simulink model "end_sem_mimuro_plot"  (R2023b)
settings: Solver=FixedStepAuto  StartTime=0.0  StopTime=20  FixedStep=0.001  RelTol=1e-3
undefined symbols (not defined in the file): simscape, X, Y, Z
libraries: sm_lib x108, nesl_utility x77, fl_lib x23, sdl_lib x5, sharedtransform x4
(part 4 of 6)

== system end_sem_mimuro_plot/Tire RL ==
  Cylindrical Solid : sm_lib/Body Elements/Cylindrical Solid  Commented=on  GraphicAmbientColor=[0.15 0.15 0.15 1.0]  BasedOnType=Density  CenterOfMass=[0 0 0]  CenterOfMassUnits=m  GraphicDiffuseColor=[0.5 0.5 0.5]  CylinderLength=0.21  CylinderLengthUnits=m  CylinderRadius=0.345  CylinderRadiusUnits=m  Density=1000  DensityUnits=kg/m^3  DoExposeReferenceFrame=on  GraphicEmissiveColor=[0.0 0.0 0.0 1.0]  ExportEntireGeometry=off  SerializedFrames=<Frames/>  MarkerShape=Sphere  MarkerSize=10  GraphicType=FromGeometry  InertiaType=Custom  Mass=20  MassUnits=kg  MomentsOfInertia=[1 2 1]  MomentsOfInertiaUnits=kg*m^2  GraphicOpacity=1.0  ProductsOfInertia=[0 0 0]  ProductsOfInertiaUnits=kg*m^2  GraphicShininess=75  GraphicSpecularColor=[0.5 0.5 0.5 1.0]  GraphicVisPropType=SimpleVisualProperties
  Inertia : sm_lib/Body Elements/Inertia  InertiaType=Custom  Mass=20  MassUnits=kg  CenterOfMass=[0 0 0]  CenterOfMassUnits=m  MomentsOfInertia=[1 2 1]  MomentsOfInertiaUnits=kg*m^2  ProductsOfInertia=[0 0 0]  ProductsOfInertiaUnits=kg*m^2  GraphicType=Marker  MarkerShape=Frame  MarkerSize=50  GraphicVisPropType=SimpleVisualProperties  GraphicDiffuseColor=[1 1 0.06667]  GraphicSpecularColor=[0.5 0.5 0.5 1.0]  GraphicAmbientColor=[0.15 0.15 0.15 1.0]  GraphicEmissiveColor=[0.0 0.0 0.0 1.0]  GraphicShininess=75  GraphicOpacity=1.0
  Tire : sm_lib/Forces and Torques/Magic Formula Tire Force and Torque  TireSide=Left  TireParameters=simscape.multibody.tirread('sm_car_heave_roll_tire_245_60_R16.tir')  SlipMode=Combined  NumericParameters=[0.1 0.1 0.1 0.1 5.0 1e-4 1e-4 1e-7 1e-7 1e-4 1e-4 0.1 1e-4 1e-4 1e-4 1e-4 1e-4 1e-4 1e-4 1e-4 1e-4]  ScalingCoefficientLMUXMode=FromTireParameters  ScalingCoefficientLMUYMode=FromTireParameters  SenseContactSignal=off  TireWrenchFrame=ContactFrame  SenseTireForce=off  SenseTireTorque=off  SensePneumaticTrail=off  SenseLongitudinalSlip=off  SenseSaturatedLongitudinalSlip=off  SenseSlipAngle=off  SenseSaturatedSlipAngle=off  SenseTurnSlip=off  SenseRelativeLongitudinalVelocity=off  SenseRelativeLateralVelocity=off  SenseLongitudinalSlipVelocity=off  SenseLateralSlipVelocity=off  SenseYawVelocity=off  SenseCamberAngle=off  SenseSaturatedCamberAngle=off  SenseCamberVelocity=off  SenseSpinVelocity=off  SenseFreeRadius=off  SenseLoadedRadius=off  SenseEffectiveRollingRadius=off  SenseLongitudinalFrictionCoefficient=off  SenseLateralFrictionCoefficient=off  SenseContactBaseRotation=off  SenseContactBaseTranslation=off  SenseContactFollowerRotation=off  SenseContactFollowerTranslation=off
  Tire Visual : Subsystem  mask(Tire Visual){tireWidth=245, aspectRatio=60, rimDia=16, rimWidth=0.205, box_color=[0.2,0.2,0.2], pulley_clr=[199,182,123]/255, box_opc=1, pulley_opc=1, lr=Left, b=9, ir=0.1, hr=0.035}
      mask prompts: rimWidth "Rim width (m)"; box_color "Tire color"; pulley_clr "Rim Color"; box_opc "Tire opacity"; pulley_opc "Rim opacity"; lr "Left/Right"; b "No. of spokes"; ir "Inner radius (m)"; hr "Hole radius (m)"
      mask init: same as end_sem_mimuro_plot/Tire FL/Tire Visual
      mask TypeOptions lr: Left | Right
      mask DialogControl ParameterGroupVar Prompt: Tire size
      mask DialogControl Control2 Prompt: /
      mask DialogControl Control3 Prompt: R
      mask DialogControl Container3 Prompt: Visual appearance
      mask DialogControl Container4 Prompt: Rim
      mask Display:
      | try
      |     image('wheel_no_brake.png')
      | catch ME
      |     fprintf('TireVisual\n')
      | end
      | 
      | % text(5,90,'Parametric Wheel Visual')
      | % f = 60;
      | % fx = 70;
      | % fx0 = 25;
      | % fy = 70;
      | % fy0 = 10;
      | % plot(-fx0+fx.*[0.8828 0.8769 0.8597 0.7299 0.7043 0.6745 0.6443 0.6195 0.5884 0.5712 0.5653 0.5573 0.5346 0.4985 0.4515 0.3965 0.3373 ]+160/2-0.43*f,-fy0+fy.*[0.3654 0.3482 0.3335 0.2583 0.2486 0.2453 0.2486 0.2583 0.2764 0.2911 0.3083 0.2449 0.1945 0.1609 0.1462 0.1520 0.1768 ]+0.3*f)
      | % plot(-fx0+fx.*[0.3255 0.3889 0.3965 0.4112 0.4313 0.3767 ]+160/2-0.43*f,-fy0+fy.*[0.1491 0.1222 0.1520 0.1777 0.1949 0.2184 ]+0.3*f)
      | % plot(-fx0+fx.*[0.3553 0.4112 0.4633 0.4826 0.5464 ]+160/2-0.43*f,-fy0+fy.*[0.2012 0.1777 0.1722 0.1898 0.2268 ]+0.3*f)
      | % plot(-fx0+fx.*[0.5426 0.5262 0.4826 0.4313 0.5603 0.5603 0.5065 ]+160/2-0.43*f,-fy0+fy.*[0.2184 0.2037 0.1898 0.1949 0.2692 0.2701 0.2932 ]+0.3*f)
      | % plot(-fx0+fx.*[0.5279 0.5460 0.4868 ]+160/2-0.43*f,-fy0+fy.*[0.3007 0.2969 0.3402 ]+0.3*f)
      | % plot(-fx0+fx.*[0.5279 0.5624 ]+160/2-0.43*f,-fy0+fy.*[0.3007 0.2856 ]+0.3*f)
      | % plot(-fx0+fx.*[0.5628 0.5460 ]+160/2-0.43*f,-fy0+fy.*[0.2898 0.2969 ]+0.3*f)
      | % plot(-fx0+fx.*[0.5712 0.5628 0.5573 ]+160/2-0.43*f,-fy0+fy.*[0.2911 0.2222 0.2449 ]+0.3*f)
      | % plot(-fx0+fx.*[0.5586 0.5422 0.5082 0.4633 0.4515 0.4481 0.3889 0.3902 0.4544 0.5099 0.5523 0.5792 0.5884 ]+160/2-0.43*f,-fy0+fy.*[0.2541 0.2180 0.1861 0.1722 0.1462 0.1163 0.1222 0.0928 0.0865 0.1033 0.1428 0.2016 0.2764 ]+0.3*f)
      | % plot(-fx0+fx.*[0.6195 0.6090 0.5792 0.5628 0.5380 0.5346 0.5422 ]+160/2-0.43*f,-fy0+fy.*[0.2583 0.1751 0.2016 0.2222 0.1680 0.1945 0.2180 ]+0.3*f)
      | % plot(-fx0+fx.*[0.5262 0.5082 0.4985 0.4994 0.5380 0.5523 0.5792 0.6090 0.6333 0.6443 ]+160/2-0.43*f,-fy0+fy.*[0.2037 0.1861 0.1609 0.1319 0.1680 0.1428 0.1092 0.1751 0.1596 0.2486 ]+0.3*f)
      | % plot(-fx0+fx.*[0.6745 0.6627 0.6333 0.6018 0.5792 0.5317 0.5099 0.4994 0.4481 0.4544 0.4700 0.5317 0.5510 0.6018 0.6291 0.6627 0.6926 0.7043 ]+160/2-0.43*f,-fy0+fy.*[0.2453 0.1508 0.1596 0.0890 0.1092 0.0655 0.1033 0.1319 0.1163 0.0865 0.0462 0.0655 0.0416 0.0890 0.0764 0.1508 0.1508 0.2486 ]+0.3*f)
      | % plot(-fx0+fx.*[0.7299 0.7178 0.6926 0.6577 0.6291 0.5758 0.5510 0.4851 0.4700 0.3986 0.3213 0.2440 0.1718 0.1100 0.0626 ]+160/2-0.43*f,-fy0+fy.*[0.2583 0.1596 0.1508 0.0739 0.0764 0.0269 0.0416 0.0210 0.0462 0.0533 0.0861 0.1424 0.2184 0.3087 0.4074 ]+0.3*f)
      | % plot(-fx0+fx.*[0.0487 0.0995 0.1100 0.1323 0.1516 0.1760 0.1399 ]+160/2-0.43*f,-fy0+fy.*[0.4082 0.3028 0.3087 0.3213 0.3326 0.3469 0.4221 ]+0.3*f)
      | % plot(-fx0+fx.*[0.1126 0.1516 0.2024 0.2234 0.2474 0.2709 0.4011 0.4200 0.4322 0.3847 0.3486 0.3255 ]+160/2-0.43*f,-fy0+fy.*[0.4141 0.3326 0.2579 0.2776 0.2969 0.3121 0.3872 0.3965 0.3982 0.4670 0.5426 0.6191 ]+0.3*f)
      | % plot(-fx0+fx.*[0.3486 0.3410 0.3755 0.3847 ]+160/2-0.43*f,-fy0+fy.*[0.5426 0.5330 0.4616 0.4670 ]+0.3*f)
      | % plot(-fx0+fx.*[0.3755 0.3570 0.3234 ]+160/2-0.43*f,-fy0+fy.*[0.4616 0.4511 0.5212 ]+0.3*f)
      | % plot(-fx0+fx.*[0.3570 0.2272 0.1936 ]+160/2-0.43*f,-fy0+fy.*[0.4511 0.3759 0.4460 ]+0.3*f)
      | % plot(-fx0+fx.*[0.1684 0.2029 0.2272 0.2709 0.3217 0.4519 0.4721 0.4868 0.4322 ]+160/2-0.43*f,-fy0+fy.*[0.4334 0.3625 0.3759 0.3121 0.2583 0.3331 0.3415 0.3402 0.3982 ]+0.3*f)
      | % plot(-fx0+fx.*[0.4200 0.3755 ]+160/2-0.43*f,-fy0+fy.*[0.3965 0.4616 ]+0.3*f)
      | % plot(-fx0+fx.*[0.3570 0.4011 0.4519 0.5065 0.5279 0.4721 0.4200 ]+160/2-0.43*f,-fy0+fy.*[0.4511 0.3872 0.3331 0.2932 0.3007 0.3415 0.3965 ]+0.3*f)
      | % plot(-fx0+fx.*[0.5065 0.3767 0.3217 0.2995 0.2474 0.2029 0.1760 0.2234 0.2785 0.2995 0.3553 0.3767 ]+160/2-0.43*f,-fy0+fy.*[0.2932 0.2184 0.2583 0.2419 0.2969 0.3625 0.3469 0.2776 0.2197 0.2419 0.2012 0.2184 ]+0.3*f)
      | % plot(-fx0+fx.*[0.3553 0.3373 0.2785 0.2617 0.2024 0.1873 0.1323 0.0899 0.0630 0.0542 0.0231 0.0059 0.0000 0.0113 0.0168 0.0332 0.0630 0.0878 0.1172 0.1470 0.1722 0.3024 0.3192 0.3255 0.3179 0.3121 0.2948 0.1651 0.1394 0.1470 0.1172 0.0878 0.0630 0.0332 0.0168 0.0113 0.0000 ]+160/2-0.43*f,-fy0+fy.*[0.2012 0.1768 0.2197 0.1957 0.2579 0.2402 0.3213 0.4099 0.4994 0.5846 0.6027 0.6174 0.6346 0.5271 0.5157 0.5078 0.4994 0.4964 0.4990 0.5061 0.5174 0.5922 0.6056 0.6191 0.6917 0.6745 0.6598 0.5846 0.5745 0.6350 0.6350 0.6434 0.6594 0.6858 0.7064 0.7291 0.6346 ]+0.3*f)
      | % plot(-fx0+fx.*[0.0059 0.0168 ]+160/2-0.43*f,-fy0+fy.*[0.6174 0.7064 ]+0.3*f)
      | % plot(-fx0+fx.*[0.0113 0.0454 0.0529 0.0181 0.0113 ]+160/2-0.43*f,-fy0+fy.*[0.7291 0.8034 0.8270 0.7497 0.7291 ]+0.3*f)
      | % plot(-fx0+fx.*[0.0168 0.0487 0.0454 ]+160/2-0.43*f,-fy0+fy.*[0.7064 0.7770 0.8034 ]+0.3*f)
      | % plot(-fx0+fx.*[0.0487 0.0626 0.0899 0.0630 0.0542 0.0794 0.0878 0.1126 0.0899 ]+160/2-0.43*f,-fy0+fy.*[0.7770 0.7518 0.7182 0.6594 0.5846 0.5745 0.6434 0.6976 0.7182 ]+0.3*f)
      | % plot(-fx0+fx.*[0.1126 0.1399 0.1684 0.1936 0.2570 ]+160/2-0.43*f,-fy0+fy.*[0.6976 0.6854 0.6829 0.6905 0.7274 ]+0.3*f)
      | % plot(-fx0+fx.*[0.3011 0.1722 0.1936 ]+160/2-0.43*f,-fy0+fy.*[0.7182 0.6438 0.6905 ]+0.3*f)
      | % plot(-fx0+fx.*[0.1684 0.1470 0.1722 0.1651 0.1722 0.1936 0.3234 0.3410 0.3192 0.3121 0.3163 ]+160/2-0.43*f,-fy0+fy.*[0.6829 0.6350 0.6438 0.5846 0.5174 0.4460 0.5212 0.5330 0.6056 0.6745 0.7119 ]+0.3*f)
      | % plot(-fx0+fx.*[0.3200 0.3179 ]+160/2-0.43*f,-fy0+fy.*[0.7102 0.6917 ]+0.3*f)
      | % plot(-fx0+fx.*[0.3020 0.2948 0.3024 0.3234 ]+160/2-0.43*f,-fy0+fy.*[0.7178 0.6598 0.5922 0.5212 ]+0.3*f)
      | % plot(-fx0+fx.*[0.1470 0.1394 0.1096 0.1172 0.1399 0.1760 0.1516 0.1323 0.1100 0.0995 0.0987 0.1688 0.1806 0.1999 0.3297 0.2566 0.1264 0.0701 0.0529 0.1084 0.1264 0.1999 ]+160/2-0.43*f,-fy0+fy.*[0.5061 0.5745 0.5716 0.6350 0.6854 0.7190 0.7341 0.7577 0.7959 0.8240 0.8530 0.8748 0.9005 0.9185 0.9933 0.9706 0.8958 0.8438 0.8270 0.8782 0.8958 0.9185 ]+0.3*f)
      | % plot(-fx0+fx.*[0.1806 0.1084 0.0987 0.0454 ]+160/2-0.43*f,-fy0+fy.*[0.9005 0.8782 0.8530 0.8034 ]+0.3*f)
      | % plot(-fx0+fx.*[0.0487 0.0995 0.1655 0.1688 ]+160/2-0.43*f,-fy0+fy.*[0.7770 0.8240 0.8446 0.8748 ]+0.3*f)
      | % plot(-fx0+fx.*[0.1655 0.1718 0.1873 0.2024 0.2234 0.2474 0.2029 0.1760 0.2234 ]+160/2-0.43*f,-fy0+fy.*[0.8446 0.8148 0.7745 0.7497 0.7333 0.7283 0.7144 0.7190 0.7333 ]+0.3*f)
      | % plot(-fx0+fx.*[0.2272 0.2478 ]+160/2-0.43*f,-fy0+fy.*[0.7215 0.7278 ]+0.3*f)
      | % plot(-fx0+fx.*[0.2272 0.2029 0.1684 ]+160/2-0.43*f,-fy0+fy.*[0.7215 0.7144 0.6829 ]+0.3*f)
      | % plot(-fx0+fx.*[0.1936 0.2272 ]+160/2-0.43*f,-fy0+fy.*[0.6905 0.7215 ]+0.3*f)
      | % plot(-fx0+fx.*[0.2024 0.1516 0.1126 ]+160/2-0.43*f,-fy0+fy.*[0.7497 0.7341 0.6976 ]+0.3*f)
      | % plot(-fx0+fx.*[0.0899 0.1323 0.1873 0.2520 0.2440 0.2428 0.2499 0.2650 0.2852 0.4150 0.4372 0.3528 0.3297 0.4150 0.5065 0.5279 0.5460 0.4586 0.4372 0.5279 ]+160/2-0.43*f,-fy0+fy.*[0.7182 0.7577 0.7745 0.7686 0.8076 0.8370 0.8669 0.8925 0.9097 0.9849 0.9920 1.0000 0.9933 0.9849 0.9458 0.9534 0.9500 0.9870 0.9920 0.9534 ]+0.3*f)
      | % plot(-fx0+fx.*[0.5065 0.3767 0.2852 0.1999 ]+160/2-0.43*f,-fy0+fy.*[0.9458 0.8711 0.9097 0.9185 ]+0.3*f)
      | % plot(-fx0+fx.*[0.1806 0.2650 0.3553 0.3767 ]+160/2-0.43*f,-fy0+fy.*[0.9005 0.8925 0.8538 0.8711 ]+0.3*f)
      | % plot(-fx0+fx.*[0.3553 0.3373 0.2499 0.1688 ]+160/2-0.43*f,-fy0+fy.*[0.8538 0.8295 0.8669 0.8748 ]+0.3*f)
      | % plot(-fx0+fx.*[0.1655 0.2428 0.3255 0.3373 ]+160/2-0.43*f,-fy0+fy.*[0.8446 0.8370 0.8018 0.8295 ]+0.3*f)
      | % plot(-fx0+fx.*[0.3255 0.3213 0.3213 0.3255 0.3373 0.2785 0.2617 0.3255 ]+160/2-0.43*f,-fy0+fy.*[0.8018 0.7749 0.7388 0.7165 0.7031 0.7278 0.7438 0.7165 ]+0.3*f)
      | % plot(-fx0+fx.*[0.3213 0.2520 0.2617 0.2024 ]+160/2-0.43*f,-fy0+fy.*[0.7388 0.7686 0.7438 0.7497 ]+0.3*f)
      | % plot(-fx0+fx.*[0.2234 0.2785 ]+160/2-0.43*f,-fy0+fy.*[0.7333 0.7278 ]+0.3*f)
      | % plot(-fx0+fx.*[0.2869 0.2474 ]+160/2-0.43*f,-fy0+fy.*[0.7241 0.7283 ]+0.3*f)
      | % plot(-fx0+fx.*[0.2440 0.3213 0.3986 0.4078 0.4246 0.4456 0.4683 0.5981 0.6182 0.6329 0.5460 ]+160/2-0.43*f,-fy0+fy.*[0.8076 0.7749 0.7186 0.7417 0.7661 0.7879 0.8043 0.8790 0.8874 0.8862 0.9500 ]+0.3*f)
      | % plot(-fx0+fx.*[0.5279 0.6182 0.7022 0.7140 0.6329 ]+160/2-0.43*f,-fy0+fy.*[0.9534 0.8874 0.7984 0.8001 0.8862 ]+0.3*f)
      | % plot(-fx0+fx.*[0.5981 0.5065 ]+160/2-0.43*f,-fy0+fy.*[0.8790 0.9458 ]+0.3*f)
      | % plot(-fx0+fx.*[0.5981 0.6829 0.7022 ]+160/2-0.43*f,-fy0+fy.*[0.8790 0.7892 0.7984 ]+0.3*f)
      | % plot(-fx0+fx.*[0.6829 0.5535 0.4683 0.3767 ]+160/2-0.43*f,-fy0+fy.*[0.7892 0.7144 0.8043 0.8711 ]+0.3*f)
      | % plot(-fx0+fx.*[0.3553 0.4456 0.5300 0.5535 ]+160/2-0.43*f,-fy0+fy.*[0.8538 0.7879 0.6989 0.7144 ]+0.3*f)
      | % plot(-fx0+fx.*[0.5300 0.5061 0.4246 0.3373 ]+160/2-0.43*f,-fy0+fy.*[0.6989 0.6800 0.7661 0.8295 ]+0.3*f)
      | % plot(-fx0+fx.*[0.3255 0.4078 0.4851 0.5061 ]+160/2-0.43*f,-fy0+fy.*[0.8018 0.7417 0.6602 0.6800 ]+0.3*f)
      | % plot(-fx0+fx.*[0.4851 0.4700 0.3986 0.3902 0.3889 0.4481 0.4544 0.4700 ]+160/2-0.43*f,-fy0+fy.*[0.6602 0.6426 0.7186 0.6884 0.6703 0.6077 0.6203 0.6426 ]+0.3*f)
      | % plot(-fx0+fx.*[0.4851 0.5510 0.5758 0.6027 0.6262 0.7560 0.7745 0.7841 0.7140 ]+160/2-0.43*f,-fy0+fy.*[0.6602 0.5632 0.5779 0.5930 0.6069 0.6816 0.6926 0.6980 0.8001 ]+0.3*f)
      | % plot(-fx0+fx.*[0.7022 0.7745 ]+160/2-0.43*f,-fy0+fy.*[0.7984 0.6926 ]+0.3*f)
      | % plot(-fx0+fx.*[0.7841 0.8375 0.8303 0.7745 ]+160/2-0.43*f,-fy0+fy.*[0.6980 0.5863 0.5766 0.6926 ]+0.3*f)
      | % plot(-fx0+fx.*[0.7560 0.6829 ]+160/2-0.43*f,-fy0+fy.*[0.6816 0.7892 ]+0.3*f)
      | % plot(-fx0+fx.*[0.7560 0.8123 0.8303 ]+160/2-0.43*f,-fy0+fy.*[0.6816 0.5649 0.5766 ]+0.3*f)
      | % plot(-fx0+fx.*[0.8123 0.6825 0.6262 0.5535 ]+160/2-0.43*f,-fy0+fy.*[0.5649 0.4901 0.6069 0.7144 ]+0.3*f)
      | % plot(-fx0+fx.*[0.5300 0.6027 0.6577 0.6825 ]+160/2-0.43*f,-fy0+fy.*[0.6989 0.5930 0.4775 0.4901 ]+0.3*f)
      | % plot(-fx0+fx.*[0.6577 0.6291 0.5758 0.5061 ]+160/2-0.43*f,-fy0+fy.*[0.4775 0.4658 0.5779 0.6800 ]+0.3*f)
      | % plot(-fx0+fx.*[0.4700 0.5317 0.5510 0.6018 0.6291 ]+160/2-0.43*f,-fy0+fy.*[0.6426 0.5523 0.5632 0.4578 0.4658 ]+0.3*f)
      | % plot(-fx0+fx.*[0.6018 0.5792 0.5317 0.5099 0.4544 0.3902 0.3213 ]+160/2-0.43*f,-fy0+fy.*[0.4578 0.4536 0.5523 0.5397 0.6203 0.6884 0.7388 ]+0.3*f)
      | % plot(-fx0+fx.*[0.3255 0.3889 0.3965 0.4515 0.4481 0.4994 0.5099 0.5523 0.5792 ]+160/2-0.43*f,-fy0+fy.*[0.7165 0.6703 0.6602 0.6018 0.6077 0.5334 0.5397 0.4511 0.4536 ]+0.3*f)
      | % plot(-fx0+fx.*[0.6018 0.6333 0.6627 0.6926 0.7178 0.8475 0.8652 0.8711 0.8375 ]+160/2-0.43*f,-fy0+fy.*[0.4578 0.3503 0.3524 0.3599 0.3713 0.4460 0.4595 0.4729 0.5863 ]+0.3*f)
      | % plot(-fx0+fx.*[0.8303 0.8652 ]+160/2-0.43*f,-fy0+fy.*[0.5766 0.4595 ]+0.3*f)
      | % plot(-fx0+fx.*[0.8711 0.8828 0.8711 0.8652 0.8475 0.7178 0.6825 0.6577 0.6027 0.5758 0.5061 0.4851 0.4078 0.3986 0.3902 0.3213 0.2520 0.1873 0.1718 0.1655 0.0995 0.0987 0.1688 0.1655 0.2428 0.2440 0.2520 0.2617 0.3255 0.3373 ]+160/2-0.43*f,-fy0+fy.*[0.4729 0.3654 0.2713 0.2503 0.2348 0.1596 0.0815 0.0739 0.0223 0.0269 0.0050 0.0210 0.0290 0.0533 0.0928 0.1222 0.1726 0.2402 0.2184 0.2058 0.3028 0.3020 0.1999 0.2058 0.1243 0.1424 0.1726 0.1957 0.1491 0.1768 ]+0.3*f)
      | % plot(-fx0+fx.*[0.3255 0.3213 0.3213 0.3255 0.4078 0.4246 0.5061 0.5300 0.6027 0.6262 0.6825 0.8123 0.8475 0.8597 0.8475 0.8123 ]+160/2-0.43*f,-fy0+fy.*[0.1491 0.1222 0.0861 0.0643 0.0290 0.0130 0.0050 0.0000 0.0223 0.0294 0.0815 0.1562 0.2348 0.3335 0.4460 0.5649 ]+0.3*f)
      | % plot(-fx0+fx.*[0.8652 0.8769 0.8652 0.8303 0.8123 0.7560 0.6262 0.5535 0.5300 0.4456 0.4246 0.3373 0.3255 0.2428 0.2499 0.3373 ]+160/2-0.43*f,-fy0+fy.*[0.4595 0.3482 0.2503 0.1735 0.1562 0.1046 0.0294 0.0067 0.0000 0.0084 0.0130 0.0504 0.0643 0.1243 0.1138 0.0504 ]+0.3*f)
      | % plot(-fx0+fx.*[0.0487 0.0168 0.0059 ]+160/2-0.43*f,-fy0+fy.*[0.4082 0.5157 0.6174 ]+0.3*f)
      | % plot(-fx0+fx.*[0.0231 0.0332 0.0626 0.1100 0.1718 0.2440 ]+160/2-0.43*f,-fy0+fy.*[0.6027 0.6858 0.7518 0.7959 0.8148 0.8076 ]+0.3*f)
      | % plot(-fx0+fx.*[0.3373 0.3965 ]+160/2-0.43*f,-fy0+fy.*[0.7031 0.6602 ]+0.3*f)
      | % plot(-fx0+fx.*[0.4515 0.4985 0.4994 0.5380 0.5523 0.5792 0.6090 0.6333 0.6443 ]+160/2-0.43*f,-fy0+fy.*[0.6018 0.5330 0.5334 0.4519 0.4511 0.3612 0.3532 0.3503 0.2486 ]+0.3*f)
      | % plot(-fx0+fx.*[0.6745 0.6627 0.6291 ]+160/2-0.43*f,-fy0+fy.*[0.2453 0.3524 0.4658 ]+0.3*f)
      | % plot(-fx0+fx.*[0.6577 0.6926 0.7043 ]+160/2-0.43*f,-fy0+fy.*[0.4775 0.3599 0.2486 ]+0.3*f)
      | % plot(-fx0+fx.*[0.7299 0.7178 0.6825 ]+160/2-0.43*f,-fy0+fy.*[0.2583 0.3713 0.4901 ]+0.3*f)
      | % plot(-fx0+fx.*[0.5792 0.6090 0.6195 ]+160/2-0.43*f,-fy0+fy.*[0.4536 0.3532 0.2583 ]+0.3*f)
      | % plot(-fx0+fx.*[0.5884 0.5792 0.5628 0.5380 0.5346 0.5573 0.5628 0.5712 ]+160/2-0.43*f,-fy0+fy.*[0.2764 0.3612 0.3692 0.4519 0.4578 0.3809 0.3692 0.2911 ]+0.3*f)
      | % plot(-fx0+fx.*[0.5653 0.5573 ]+160/2-0.43*f,-fy0+fy.*[0.3083 0.3809 ]+0.3*f)
      | % plot(-fx0+fx.*[0.5346 0.4985 ]+160/2-0.43*f,-fy0+fy.*[0.4578 0.5330 ]+0.3*f)
      | % plot(-fx0+fx.*[0.1470 0.1684 0.1936 ]+160/2-0.43*f,-fy0+fy.*[0.5061 0.4334 0.4460 ]+0.3*f)
      | % plot(-fx0+fx.*[0.1684 0.1399 0.1172 0.1096 0.0794 0.0878 0.1126 0.1399 ]+160/2-0.43*f,-fy0+fy.*[0.4334 0.4221 0.4990 0.5716 0.5745 0.4964 0.4141 0.4221 ]+0.3*f)
      | % plot(-fx0+fx.*[0.1126 0.0899 0.0626 0.0332 0.0231 ]+160/2-0.43*f,-fy0+fy.*[0.4141 0.4099 0.4074 0.5078 0.6027 ]+0.3*f)
      | % plot(-fx0+fx.*[0.0113 0.0454 0.0487 0.0626 ]+160/2-0.43*f,-fy0+fy.*[0.5271 0.4137 0.4082 0.4074 ]+0.3*f)
      | % plot(-fx0+fx.*[0.0454 0.0987 ]+160/2-0.43*f,-fy0+fy.*[0.4137 0.3020 ]+0.3*f)
  C : PMIOPort  Side=Left
  G : PMIOPort  Port=2  Side=Right
  connections:
  Tire/LConn1 -- G/RConn1
  Cylindrical Solid/RConn1 -- Inertia/RConn1 -- Tire Visual/LConn1 -- C/RConn1 -- Tire/RConn1

== system end_sem_mimuro_plot/Tire RR ==
  Cylindrical Solid : sm_lib/Body Elements/Cylindrical Solid  Commented=on  GraphicAmbientColor=[0.15 0.15 0.15 1.0]  BasedOnType=Density  CenterOfMass=[0 0 0]  CenterOfMassUnits=m  GraphicDiffuseColor=[0.5 0.5 0.5]  CylinderLength=0.21  CylinderLengthUnits=m  CylinderRadius=0.345  CylinderRadiusUnits=m  Density=1000  DensityUnits=kg/m^3  DoExposeReferenceFrame=on  GraphicEmissiveColor=[0.0 0.0 0.0 1.0]  ExportEntireGeometry=off  SerializedFrames=<Frames/>  MarkerShape=Sphere  MarkerSize=10  GraphicType=FromGeometry  InertiaType=Custom  Mass=20  MassUnits=kg  MomentsOfInertia=[1 2 1]  MomentsOfInertiaUnits=kg*m^2  GraphicOpacity=1.0  ProductsOfInertia=[0 0 0]  ProductsOfInertiaUnits=kg*m^2  GraphicShininess=75  GraphicSpecularColor=[0.5 0.5 0.5 1.0]  GraphicVisPropType=SimpleVisualProperties
  Inertia : sm_lib/Body Elements/Inertia  InertiaType=Custom  Mass=20  MassUnits=kg  CenterOfMass=[0 0 0]  CenterOfMassUnits=m  MomentsOfInertia=[1 2 1]  MomentsOfInertiaUnits=kg*m^2  ProductsOfInertia=[0 0 0]  ProductsOfInertiaUnits=kg*m^2  GraphicType=Marker  MarkerShape=Frame  MarkerSize=50  GraphicVisPropType=SimpleVisualProperties  GraphicDiffuseColor=[1 1 0.06667]  GraphicSpecularColor=[0.5 0.5 0.5 1.0]  GraphicAmbientColor=[0.15 0.15 0.15 1.0]  GraphicEmissiveColor=[0.0 0.0 0.0 1.0]  GraphicShininess=75  GraphicOpacity=1.0
  Tire : sm_lib/Forces and Torques/Magic Formula Tire Force and Torque  TireSide=Right  TireParameters=simscape.multibody.tirread('sm_car_heave_roll_tire_245_60_R16.tir')  SlipMode=Combined  NumericParameters=[0.1 0.1 0.1 0.1 5.0 1e-4 1e-4 1e-7 1e-7 1e-4 1e-4 0.1 1e-4 1e-4 1e-4 1e-4 1e-4 1e-4 1e-4 1e-4 1e-4]  ScalingCoefficientLMUXMode=FromTireParameters  ScalingCoefficientLMUYMode=FromTireParameters  SenseContactSignal=off  TireWrenchFrame=ContactFrame  SenseTireForce=off  SenseTireTorque=off  SensePneumaticTrail=off  SenseLongitudinalSlip=off  SenseSaturatedLongitudinalSlip=off  SenseSlipAngle=off  SenseSaturatedSlipAngle=off  SenseTurnSlip=off  SenseRelativeLongitudinalVelocity=off  SenseRelativeLateralVelocity=off  SenseLongitudinalSlipVelocity=off  SenseLateralSlipVelocity=off  SenseYawVelocity=off  SenseCamberAngle=off  SenseSaturatedCamberAngle=off  SenseCamberVelocity=off  SenseSpinVelocity=off  SenseFreeRadius=off  SenseLoadedRadius=off  SenseEffectiveRollingRadius=off  SenseLongitudinalFrictionCoefficient=off  SenseLateralFrictionCoefficient=off  SenseContactBaseRotation=off  SenseContactBaseTranslation=off  SenseContactFollowerRotation=off  SenseContactFollowerTranslation=off
  Tire Visual : Subsystem  mask(Tire Visual){tireWidth=245, aspectRatio=60, rimDia=16, rimWidth=0.205, box_color=[0.2,0.2,0.2], pulley_clr=[199,182,123]/255, box_opc=1, pulley_opc=1, lr=Left, b=9, ir=0.1, hr=0.035}
      mask prompts: rimWidth "Rim width (m)"; box_color "Tire color"; pulley_clr "Rim Color"; box_opc "Tire opacity"; pulley_opc "Rim opacity"; lr "Left/Right"; b "No. of spokes"; ir "Inner radius (m)"; hr "Hole radius (m)"
      mask init: same as end_sem_mimuro_plot/Tire FL/Tire Visual
      mask TypeOptions lr: Left | Right
      mask DialogControl ParameterGroupVar Prompt: Tire size
      mask DialogControl Control2 Prompt: /
      mask DialogControl Control3 Prompt: R
      mask DialogControl Container3 Prompt: Visual appearance
      mask DialogControl Container4 Prompt: Rim
      mask Display:
      | try
      |     image('wheel_no_brake.png')
      | catch ME
      |     fprintf('TireVisual\n')
      | end
      | 
      | % text(5,90,'Parametric Wheel Visual')
      | % f = 60;
      | % fx = 70;
      | % fx0 = 25;
      | % fy = 70;
      | % fy0 = 10;
      | % plot(-fx0+fx.*[0.8828 0.8769 0.8597 0.7299 0.7043 0.6745 0.6443 0.6195 0.5884 0.5712 0.5653 0.5573 0.5346 0.4985 0.4515 0.3965 0.3373 ]+160/2-0.43*f,-fy0+fy.*[0.3654 0.3482 0.3335 0.2583 0.2486 0.2453 0.2486 0.2583 0.2764 0.2911 0.3083 0.2449 0.1945 0.1609 0.1462 0.1520 0.1768 ]+0.3*f)
      | % plot(-fx0+fx.*[0.3255 0.3889 0.3965 0.4112 0.4313 0.3767 ]+160/2-0.43*f,-fy0+fy.*[0.1491 0.1222 0.1520 0.1777 0.1949 0.2184 ]+0.3*f)
      | % plot(-fx0+fx.*[0.3553 0.4112 0.4633 0.4826 0.5464 ]+160/2-0.43*f,-fy0+fy.*[0.2012 0.1777 0.1722 0.1898 0.2268 ]+0.3*f)
      | % plot(-fx0+fx.*[0.5426 0.5262 0.4826 0.4313 0.5603 0.5603 0.5065 ]+160/2-0.43*f,-fy0+fy.*[0.2184 0.2037 0.1898 0.1949 0.2692 0.2701 0.2932 ]+0.3*f)
      | % plot(-fx0+fx.*[0.5279 0.5460 0.4868 ]+160/2-0.43*f,-fy0+fy.*[0.3007 0.2969 0.3402 ]+0.3*f)
      | % plot(-fx0+fx.*[0.5279 0.5624 ]+160/2-0.43*f,-fy0+fy.*[0.3007 0.2856 ]+0.3*f)
      | % plot(-fx0+fx.*[0.5628 0.5460 ]+160/2-0.43*f,-fy0+fy.*[0.2898 0.2969 ]+0.3*f)
      | % plot(-fx0+fx.*[0.5712 0.5628 0.5573 ]+160/2-0.43*f,-fy0+fy.*[0.2911 0.2222 0.2449 ]+0.3*f)
      | % plot(-fx0+fx.*[0.5586 0.5422 0.5082 0.4633 0.4515 0.4481 0.3889 0.3902 0.4544 0.5099 0.5523 0.5792 0.5884 ]+160/2-0.43*f,-fy0+fy.*[0.2541 0.2180 0.1861 0.1722 0.1462 0.1163 0.1222 0.0928 0.0865 0.1033 0.1428 0.2016 0.2764 ]+0.3*f)
      | % plot(-fx0+fx.*[0.6195 0.6090 0.5792 0.5628 0.5380 0.5346 0.5422 ]+160/2-0.43*f,-fy0+fy.*[0.2583 0.1751 0.2016 0.2222 0.1680 0.1945 0.2180 ]+0.3*f)
      | % plot(-fx0+fx.*[0.5262 0.5082 0.4985 0.4994 0.5380 0.5523 0.5792 0.6090 0.6333 0.6443 ]+160/2-0.43*f,-fy0+fy.*[0.2037 0.1861 0.1609 0.1319 0.1680 0.1428 0.1092 0.1751 0.1596 0.2486 ]+0.3*f)
      | % plot(-fx0+fx.*[0.6745 0.6627 0.6333 0.6018 0.5792 0.5317 0.5099 0.4994 0.4481 0.4544 0.4700 0.5317 0.5510 0.6018 0.6291 0.6627 0.6926 0.7043 ]+160/2-0.43*f,-fy0+fy.*[0.2453 0.1508 0.1596 0.0890 0.1092 0.0655 0.1033 0.1319 0.1163 0.0865 0.0462 0.0655 0.0416 0.0890 0.0764 0.1508 0.1508 0.2486 ]+0.3*f)
      | % plot(-fx0+fx.*[0.7299 0.7178 0.6926 0.6577 0.6291 0.5758 0.5510 0.4851 0.4700 0.3986 0.3213 0.2440 0.1718 0.1100 0.0626 ]+160/2-0.43*f,-fy0+fy.*[0.2583 0.1596 0.1508 0.0739 0.0764 0.0269 0.0416 0.0210 0.0462 0.0533 0.0861 0.1424 0.2184 0.3087 0.4074 ]+0.3*f)
      | % plot(-fx0+fx.*[0.0487 0.0995 0.1100 0.1323 0.1516 0.1760 0.1399 ]+160/2-0.43*f,-fy0+fy.*[0.4082 0.3028 0.3087 0.3213 0.3326 0.3469 0.4221 ]+0.3*f)
      | % plot(-fx0+fx.*[0.1126 0.1516 0.2024 0.2234 0.2474 0.2709 0.4011 0.4200 0.4322 0.3847 0.3486 0.3255 ]+160/2-0.43*f,-fy0+fy.*[0.4141 0.3326 0.2579 0.2776 0.2969 0.3121 0.3872 0.3965 0.3982 0.4670 0.5426 0.6191 ]+0.3*f)
      | % plot(-fx0+fx.*[0.3486 0.3410 0.3755 0.3847 ]+160/2-0.43*f,-fy0+fy.*[0.5426 0.5330 0.4616 0.4670 ]+0.3*f)
      | % plot(-fx0+fx.*[0.3755 0.3570 0.3234 ]+160/2-0.43*f,-fy0+fy.*[0.4616 0.4511 0.5212 ]+0.3*f)
      | % plot(-fx0+fx.*[0.3570 0.2272 0.1936 ]+160/2-0.43*f,-fy0+fy.*[0.4511 0.3759 0.4460 ]+0.3*f)
      | % plot(-fx0+fx.*[0.1684 0.2029 0.2272 0.2709 0.3217 0.4519 0.4721 0.4868 0.4322 ]+160/2-0.43*f,-fy0+fy.*[0.4334 0.3625 0.3759 0.3121 0.2583 0.3331 0.3415 0.3402 0.3982 ]+0.3*f)
      | % plot(-fx0+fx.*[0.4200 0.3755 ]+160/2-0.43*f,-fy0+fy.*[0.3965 0.4616 ]+0.3*f)
      | % plot(-fx0+fx.*[0.3570 0.4011 0.4519 0.5065 0.5279 0.4721 0.4200 ]+160/2-0.43*f,-fy0+fy.*[0.4511 0.3872 0.3331 0.2932 0.3007 0.3415 0.3965 ]+0.3*f)
      | % plot(-fx0+fx.*[0.5065 0.3767 0.3217 0.2995 0.2474 0.2029 0.1760 0.2234 0.2785 0.2995 0.3553 0.3767 ]+160/2-0.43*f,-fy0+fy.*[0.2932 0.2184 0.2583 0.2419 0.2969 0.3625 0.3469 0.2776 0.2197 0.2419 0.2012 0.2184 ]+0.3*f)
      | % plot(-fx0+fx.*[0.3553 0.3373 0.2785 0.2617 0.2024 0.1873 0.1323 0.0899 0.0630 0.0542 0.0231 0.0059 0.0000 0.0113 0.0168 0.0332 0.0630 0.0878 0.1172 0.1470 0.1722 0.3024 0.3192 0.3255 0.3179 0.3121 0.2948 0.1651 0.1394 0.1470 0.1172 0.0878 0.0630 0.0332 0.0168 0.0113 0.0000 ]+160/2-0.43*f,-fy0+fy.*[0.2012 0.1768 0.2197 0.1957 0.2579 0.2402 0.3213 0.4099 0.4994 0.5846 0.6027 0.6174 0.6346 0.5271 0.5157 0.5078 0.4994 0.4964 0.4990 0.5061 0.5174 0.5922 0.6056 0.6191 0.6917 0.6745 0.6598 0.5846 0.5745 0.6350 0.6350 0.6434 0.6594 0.6858 0.7064 0.7291 0.6346 ]+0.3*f)
      | % plot(-fx0+fx.*[0.0059 0.0168 ]+160/2-0.43*f,-fy0+fy.*[0.6174 0.7064 ]+0.3*f)
      | % plot(-fx0+fx.*[0.0113 0.0454 0.0529 0.0181 0.0113 ]+160/2-0.43*f,-fy0+fy.*[0.7291 0.8034 0.8270 0.7497 0.7291 ]+0.3*f)
      | % plot(-fx0+fx.*[0.0168 0.0487 0.0454 ]+160/2-0.43*f,-fy0+fy.*[0.7064 0.7770 0.8034 ]+0.3*f)
      | % plot(-fx0+fx.*[0.0487 0.0626 0.0899 0.0630 0.0542 0.0794 0.0878 0.1126 0.0899 ]+160/2-0.43*f,-fy0+fy.*[0.7770 0.7518 0.7182 0.6594 0.5846 0.5745 0.6434 0.6976 0.7182 ]+0.3*f)
      | % plot(-fx0+fx.*[0.1126 0.1399 0.1684 0.1936 0.2570 ]+160/2-0.43*f,-fy0+fy.*[0.6976 0.6854 0.6829 0.6905 0.7274 ]+0.3*f)
      | % plot(-fx0+fx.*[0.3011 0.1722 0.1936 ]+160/2-0.43*f,-fy0+fy.*[0.7182 0.6438 0.6905 ]+0.3*f)
      | % plot(-fx0+fx.*[0.1684 0.1470 0.1722 0.1651 0.1722 0.1936 0.3234 0.3410 0.3192 0.3121 0.3163 ]+160/2-0.43*f,-fy0+fy.*[0.6829 0.6350 0.6438 0.5846 0.5174 0.4460 0.5212 0.5330 0.6056 0.6745 0.7119 ]+0.3*f)
      | % plot(-fx0+fx.*[0.3200 0.3179 ]+160/2-0.43*f,-fy0+fy.*[0.7102 0.6917 ]+0.3*f)
      | % plot(-fx0+fx.*[0.3020 0.2948 0.3024 0.3234 ]+160/2-0.43*f,-fy0+fy.*[0.7178 0.6598 0.5922 0.5212 ]+0.3*f)
      | % plot(-fx0+fx.*[0.1470 0.1394 0.1096 0.1172 0.1399 0.1760 0.1516 0.1323 0.1100 0.0995 0.0987 0.1688 0.1806 0.1999 0.3297 0.2566 0.1264 0.0701 0.0529 0.1084 0.1264 0.1999 ]+160/2-0.43*f,-fy0+fy.*[0.5061 0.5745 0.5716 0.6350 0.6854 0.7190 0.7341 0.7577 0.7959 0.8240 0.8530 0.8748 0.9005 0.9185 0.9933 0.9706 0.8958 0.8438 0.8270 0.8782 0.8958 0.9185 ]+0.3*f)
      | % plot(-fx0+fx.*[0.1806 0.1084 0.0987 0.0454 ]+160/2-0.43*f,-fy0+fy.*[0.9005 0.8782 0.8530 0.8034 ]+0.3*f)
      | % plot(-fx0+fx.*[0.0487 0.0995 0.1655 0.1688 ]+160/2-0.43*f,-fy0+fy.*[0.7770 0.8240 0.8446 0.8748 ]+0.3*f)
      | % plot(-fx0+fx.*[0.1655 0.1718 0.1873 0.2024 0.2234 0.2474 0.2029 0.1760 0.2234 ]+160/2-0.43*f,-fy0+fy.*[0.8446 0.8148 0.7745 0.7497 0.7333 0.7283 0.7144 0.7190 0.7333 ]+0.3*f)
      | % plot(-fx0+fx.*[0.2272 0.2478 ]+160/2-0.43*f,-fy0+fy.*[0.7215 0.7278 ]+0.3*f)
      | % plot(-fx0+fx.*[0.2272 0.2029 0.1684 ]+160/2-0.43*f,-fy0+fy.*[0.7215 0.7144 0.6829 ]+0.3*f)
      | % plot(-fx0+fx.*[0.1936 0.2272 ]+160/2-0.43*f,-fy0+fy.*[0.6905 0.7215 ]+0.3*f)
      | % plot(-fx0+fx.*[0.2024 0.1516 0.1126 ]+160/2-0.43*f,-fy0+fy.*[0.7497 0.7341 0.6976 ]+0.3*f)
      | % plot(-fx0+fx.*[0.0899 0.1323 0.1873 0.2520 0.2440 0.2428 0.2499 0.2650 0.2852 0.4150 0.4372 0.3528 0.3297 0.4150 0.5065 0.5279 0.5460 0.4586 0.4372 0.5279 ]+160/2-0.43*f,-fy0+fy.*[0.7182 0.7577 0.7745 0.7686 0.8076 0.8370 0.8669 0.8925 0.9097 0.9849 0.9920 1.0000 0.9933 0.9849 0.9458 0.9534 0.9500 0.9870 0.9920 0.9534 ]+0.3*f)
      | % plot(-fx0+fx.*[0.5065 0.3767 0.2852 0.1999 ]+160/2-0.43*f,-fy0+fy.*[0.9458 0.8711 0.9097 0.9185 ]+0.3*f)
      | % plot(-fx0+fx.*[0.1806 0.2650 0.3553 0.3767 ]+160/2-0.43*f,-fy0+fy.*[0.9005 0.8925 0.8538 0.8711 ]+0.3*f)
      | % plot(-fx0+fx.*[0.3553 0.3373 0.2499 0.1688 ]+160/2-0.43*f,-fy0+fy.*[0.8538 0.8295 0.8669 0.8748 ]+0.3*f)
      | % plot(-fx0+fx.*[0.1655 0.2428 0.3255 0.3373 ]+160/2-0.43*f,-fy0+fy.*[0.8446 0.8370 0.8018 0.8295 ]+0.3*f)
      | % plot(-fx0+fx.*[0.3255 0.3213 0.3213 0.3255 0.3373 0.2785 0.2617 0.3255 ]+160/2-0.43*f,-fy0+fy.*[0.8018 0.7749 0.7388 0.7165 0.7031 0.7278 0.7438 0.7165 ]+0.3*f)
      | % plot(-fx0+fx.*[0.3213 0.2520 0.2617 0.2024 ]+160/2-0.43*f,-fy0+fy.*[0.7388 0.7686 0.7438 0.7497 ]+0.3*f)
      | % plot(-fx0+fx.*[0.2234 0.2785 ]+160/2-0.43*f,-fy0+fy.*[0.7333 0.7278 ]+0.3*f)
      | % plot(-fx0+fx.*[0.2869 0.2474 ]+160/2-0.43*f,-fy0+fy.*[0.7241 0.7283 ]+0.3*f)
      | % plot(-fx0+fx.*[0.2440 0.3213 0.3986 0.4078 0.4246 0.4456 0.4683 0.5981 0.6182 0.6329 0.5460 ]+160/2-0.43*f,-fy0+fy.*[0.8076 0.7749 0.7186 0.7417 0.7661 0.7879 0.8043 0.8790 0.8874 0.8862 0.9500 ]+0.3*f)
      | % plot(-fx0+fx.*[0.5279 0.6182 0.7022 0.7140 0.6329 ]+160/2-0.43*f,-fy0+fy.*[0.9534 0.8874 0.7984 0.8001 0.8862 ]+0.3*f)
      | % plot(-fx0+fx.*[0.5981 0.5065 ]+160/2-0.43*f,-fy0+fy.*[0.8790 0.9458 ]+0.3*f)
      | % plot(-fx0+fx.*[0.5981 0.6829 0.7022 ]+160/2-0.43*f,-fy0+fy.*[0.8790 0.7892 0.7984 ]+0.3*f)
      | % plot(-fx0+fx.*[0.6829 0.5535 0.4683 0.3767 ]+160/2-0.43*f,-fy0+fy.*[0.7892 0.7144 0.8043 0.8711 ]+0.3*f)
      | % plot(-fx0+fx.*[0.3553 0.4456 0.5300 0.5535 ]+160/2-0.43*f,-fy0+fy.*[0.8538 0.7879 0.6989 0.7144 ]+0.3*f)
      | % plot(-fx0+fx.*[0.5300 0.5061 0.4246 0.3373 ]+160/2-0.43*f,-fy0+fy.*[0.6989 0.6800 0.7661 0.8295 ]+0.3*f)
      | % plot(-fx0+fx.*[0.3255 0.4078 0.4851 0.5061 ]+160/2-0.43*f,-fy0+fy.*[0.8018 0.7417 0.6602 0.6800 ]+0.3*f)
      | % plot(-fx0+fx.*[0.4851 0.4700 0.3986 0.3902 0.3889 0.4481 0.4544 0.4700 ]+160/2-0.43*f,-fy0+fy.*[0.6602 0.6426 0.7186 0.6884 0.6703 0.6077 0.6203 0.6426 ]+0.3*f)
      | % plot(-fx0+fx.*[0.4851 0.5510 0.5758 0.6027 0.6262 0.7560 0.7745 0.7841 0.7140 ]+160/2-0.43*f,-fy0+fy.*[0.6602 0.5632 0.5779 0.5930 0.6069 0.6816 0.6926 0.6980 0.8001 ]+0.3*f)
      | % plot(-fx0+fx.*[0.7022 0.7745 ]+160/2-0.43*f,-fy0+fy.*[0.7984 0.6926 ]+0.3*f)
      | % plot(-fx0+fx.*[0.7841 0.8375 0.8303 0.7745 ]+160/2-0.43*f,-fy0+fy.*[0.6980 0.5863 0.5766 0.6926 ]+0.3*f)
      | % plot(-fx0+fx.*[0.7560 0.6829 ]+160/2-0.43*f,-fy0+fy.*[0.6816 0.7892 ]+0.3*f)
      | % plot(-fx0+fx.*[0.7560 0.8123 0.8303 ]+160/2-0.43*f,-fy0+fy.*[0.6816 0.5649 0.5766 ]+0.3*f)
      | % plot(-fx0+fx.*[0.8123 0.6825 0.6262 0.5535 ]+160/2-0.43*f,-fy0+fy.*[0.5649 0.4901 0.6069 0.7144 ]+0.3*f)
      | % plot(-fx0+fx.*[0.5300 0.6027 0.6577 0.6825 ]+160/2-0.43*f,-fy0+fy.*[0.6989 0.5930 0.4775 0.4901 ]+0.3*f)
      | % plot(-fx0+fx.*[0.6577 0.6291 0.5758 0.5061 ]+160/2-0.43*f,-fy0+fy.*[0.4775 0.4658 0.5779 0.6800 ]+0.3*f)
      | % plot(-fx0+fx.*[0.4700 0.5317 0.5510 0.6018 0.6291 ]+160/2-0.43*f,-fy0+fy.*[0.6426 0.5523 0.5632 0.4578 0.4658 ]+0.3*f)
      | % plot(-fx0+fx.*[0.6018 0.5792 0.5317 0.5099 0.4544 0.3902 0.3213 ]+160/2-0.43*f,-fy0+fy.*[0.4578 0.4536 0.5523 0.5397 0.6203 0.6884 0.7388 ]+0.3*f)
      | % plot(-fx0+fx.*[0.3255 0.3889 0.3965 0.4515 0.4481 0.4994 0.5099 0.5523 0.5792 ]+160/2-0.43*f,-fy0+fy.*[0.7165 0.6703 0.6602 0.6018 0.6077 0.5334 0.5397 0.4511 0.4536 ]+0.3*f)
      | % plot(-fx0+fx.*[0.6018 0.6333 0.6627 0.6926 0.7178 0.8475 0.8652 0.8711 0.8375 ]+160/2-0.43*f,-fy0+fy.*[0.4578 0.3503 0.3524 0.3599 0.3713 0.4460 0.4595 0.4729 0.5863 ]+0.3*f)
      | % plot(-fx0+fx.*[0.8303 0.8652 ]+160/2-0.43*f,-fy0+fy.*[0.5766 0.4595 ]+0.3*f)
      | % plot(-fx0+fx.*[0.8711 0.8828 0.8711 0.8652 0.8475 0.7178 0.6825 0.6577 0.6027 0.5758 0.5061 0.4851 0.4078 0.3986 0.3902 0.3213 0.2520 0.1873 0.1718 0.1655 0.0995 0.0987 0.1688 0.1655 0.2428 0.2440 0.2520 0.2617 0.3255 0.3373 ]+160/2-0.43*f,-fy0+fy.*[0.4729 0.3654 0.2713 0.2503 0.2348 0.1596 0.0815 0.0739 0.0223 0.0269 0.0050 0.0210 0.0290 0.0533 0.0928 0.1222 0.1726 0.2402 0.2184 0.2058 0.3028 0.3020 0.1999 0.2058 0.1243 0.1424 0.1726 0.1957 0.1491 0.1768 ]+0.3*f)
      | % plot(-fx0+fx.*[0.3255 0.3213 0.3213 0.3255 0.4078 0.4246 0.5061 0.5300 0.6027 0.6262 0.6825 0.8123 0.8475 0.8597 0.8475 0.8123 ]+160/2-0.43*f,-fy0+fy.*[0.1491 0.1222 0.0861 0.0643 0.0290 0.0130 0.0050 0.0000 0.0223 0.0294 0.0815 0.1562 0.2348 0.3335 0.4460 0.5649 ]+0.3*f)
      | % plot(-fx0+fx.*[0.8652 0.8769 0.8652 0.8303 0.8123 0.7560 0.6262 0.5535 0.5300 0.4456 0.4246 0.3373 0.3255 0.2428 0.2499 0.3373 ]+160/2-0.43*f,-fy0+fy.*[0.4595 0.3482 0.2503 0.1735 0.1562 0.1046 0.0294 0.0067 0.0000 0.0084 0.0130 0.0504 0.0643 0.1243 0.1138 0.0504 ]+0.3*f)
      | % plot(-fx0+fx.*[0.0487 0.0168 0.0059 ]+160/2-0.43*f,-fy0+fy.*[0.4082 0.5157 0.6174 ]+0.3*f)
      | % plot(-fx0+fx.*[0.0231 0.0332 0.0626 0.1100 0.1718 0.2440 ]+160/2-0.43*f,-fy0+fy.*[0.6027 0.6858 0.7518 0.7959 0.8148 0.8076 ]+0.3*f)
      | % plot(-fx0+fx.*[0.3373 0.3965 ]+160/2-0.43*f,-fy0+fy.*[0.7031 0.6602 ]+0.3*f)
      | % plot(-fx0+fx.*[0.4515 0.4985 0.4994 0.5380 0.5523 0.5792 0.6090 0.6333 0.6443 ]+160/2-0.43*f,-fy0+fy.*[0.6018 0.5330 0.5334 0.4519 0.4511 0.3612 0.3532 0.3503 0.2486 ]+0.3*f)
      | % plot(-fx0+fx.*[0.6745 0.6627 0.6291 ]+160/2-0.43*f,-fy0+fy.*[0.2453 0.3524 0.4658 ]+0.3*f)
      | % plot(-fx0+fx.*[0.6577 0.6926 0.7043 ]+160/2-0.43*f,-fy0+fy.*[0.4775 0.3599 0.2486 ]+0.3*f)
      | % plot(-fx0+fx.*[0.7299 0.7178 0.6825 ]+160/2-0.43*f,-fy0+fy.*[0.2583 0.3713 0.4901 ]+0.3*f)
      | % plot(-fx0+fx.*[0.5792 0.6090 0.6195 ]+160/2-0.43*f,-fy0+fy.*[0.4536 0.3532 0.2583 ]+0.3*f)
      | % plot(-fx0+fx.*[0.5884 0.5792 0.5628 0.5380 0.5346 0.5573 0.5628 0.5712 ]+160/2-0.43*f,-fy0+fy.*[0.2764 0.3612 0.3692 0.4519 0.4578 0.3809 0.3692 0.2911 ]+0.3*f)
      | % plot(-fx0+fx.*[0.5653 0.5573 ]+160/2-0.43*f,-fy0+fy.*[0.3083 0.3809 ]+0.3*f)
      | % plot(-fx0+fx.*[0.5346 0.4985 ]+160/2-0.43*f,-fy0+fy.*[0.4578 0.5330 ]+0.3*f)
      | % plot(-fx0+fx.*[0.1470 0.1684 0.1936 ]+160/2-0.43*f,-fy0+fy.*[0.5061 0.4334 0.4460 ]+0.3*f)
      | % plot(-fx0+fx.*[0.1684 0.1399 0.1172 0.1096 0.0794 0.0878 0.1126 0.1399 ]+160/2-0.43*f,-fy0+fy.*[0.4334 0.4221 0.4990 0.5716 0.5745 0.4964 0.4141 0.4221 ]+0.3*f)
      | % plot(-fx0+fx.*[0.1126 0.0899 0.0626 0.0332 0.0231 ]+160/2-0.43*f,-fy0+fy.*[0.4141 0.4099 0.4074 0.5078 0.6027 ]+0.3*f)
      | % plot(-fx0+fx.*[0.0113 0.0454 0.0487 0.0626 ]+160/2-0.43*f,-fy0+fy.*[0.5271 0.4137 0.4082 0.4074 ]+0.3*f)
      | % plot(-fx0+fx.*[0.0454 0.0987 ]+160/2-0.43*f,-fy0+fy.*[0.4137 0.3020 ]+0.3*f)
  C : PMIOPort  Side=Left
  G : PMIOPort  Port=2  Side=Right
  connections:
  Tire/RConn1 -- C/RConn1 -- Tire Visual/LConn1 -- Inertia/RConn1 -- Cylindrical Solid/RConn1
  Tire/LConn1 -- G/RConn1

== system end_sem_mimuro_plot/body visual ==
  Extruded Solid : sm_lib/Body Elements/Extruded Solid  GraphicAmbientColor=[0.15 0.15 0.15 1.0]  BasedOnType=Density  CenterOfMass=[0 0 0]  CenterOfMassUnits=m  GraphicDiffuseColor=[0.0 0.49803922 0.49803922]  ExportConvexHullGeometry=off  ExtrusionCrossSection=cs1  ExtrusionCrossSectionUnits=m  Density=0.001  DensityUnits=kg/m^3  DoExposeReferenceFrame=on  GraphicEmissiveColor=[0.0 0.0 0.0 1.0]  ExportEntireGeometry=off  ExtrusionLength=0.8  ExtrusionLengthUnits=m  ExtrusionType=General  SerializedFrames=<Frames/>  MarkerShape=Sphere  MarkerSize=10  GraphicType=FromGeometry  InertiaType=CalculateFromGeometry  Mass=1  MassUnits=kg  MomentsOfInertia=[1 1 1]  MomentsOfInertiaUnits=kg*m^2  PolygonNumSides=3  GraphicOpacity=0.35  PolygonOuterRadius=1  PolygonOuterRadiusUnits=m  ProductsOfInertia=[0 0 0]  ProductsOfInertiaUnits=kg*m^2  GraphicShininess=75  GraphicSpecularColor=[0.5 0.5 0.5 1.0]  GraphicVisPropType=SimpleVisualProperties
  Rigid Transform : sm_lib/Frames and Transforms/Rigid Transform  TranslationMethod=Cartesian  TranslationStandardOffset=0  TranslationStandardOffsetUnits=m  TranslationStandardAxis=+Z  TranslationCartesianOffset=[0.35 0 0]  TranslationCartesianOffsetUnits=m  TranslationROffset=0  TranslationROffsetUnits=m  TranslationZOffset=0  TranslationZOffsetUnits=m  TranslationThetaOffset=0  TranslationThetaOffsetUnits=deg  RotationMethod=StandardAxis  RotationAngleUnits=deg  RotationStandardAxis=+X  RotationAngle=90  RotationArbitraryAxis=[0 0 1]  FollAlignAxisA=+X  BaseAlignAxisA=+Y  FollAlignAxisB=+Y  BaseAlignAxisB=+Z  RotationSequenceAxes=FollowerAxes  RotationSequence=XYX  RotationSequenceAngles=[0 0 0]  RotationSequenceAnglesUnits=deg  RotationMatrix=[1 0 0; 0 1 0; 0 0 1]  Quaternion=[1 0 0 0]
  C : PMIOPort  Side=Left
  connections:
  Rigid Transform/LConn1 -- C/RConn1
  Extruded Solid/RConn1 -- Rigid Transform/RConn1

== system end_sem_mimuro_plot/6 DOF/Tx Sensor ==
  Bus Creator : BusCreator  Inputs=12
  Transform Sensor : sm_lib/Frames and Transforms/Transform Sensor  Commented=on  MeasurementFrame=World  RotationSequence=XYX  SenseAngle=off  SenseAxis=off  SenseQ=off  SenseR=off  SenseRotationSequence=off  SenseOmegaX=off  SenseOmegaY=off  SenseOmegaZ=off  SenseOmega=off  SenseQDot=off  SenseRDot=off  SenseRotationSequenceDot=off  SenseAlphaX=off  SenseAlphaY=off  SenseAlphaZ=off  SenseAlpha=off  SenseQDDot=off  SenseRDDot=off  SenseX=off  SenseY=off  SenseZ=off  SenseXYZ=off  SenseRad=off  SenseAzim=off  SenseDist=off  SenseInc=off  SenseXDot=off  SenseYDot=off  SenseZDot=off  SenseXYZDot=off  SenseRadDot=off  SenseAzimDot=off  SenseDistDot=off  SenseIncDot=off  SenseXDDot=off  SenseYDDot=off  SenseZDDot=off  SenseXYZDDot=off  SenseRadDDot=off  SenseAzimDDot=off  SenseDistDDot=off  SenseIncDDot=off
  World Frame : sm_lib/Frames and Transforms/World Frame
  non rotating follower - vehicle frame : Subsystem
  world frame : Subsystem
  F : PMIOPort  Side=Right
  S : Outport
  wires:
  Bus Creator/1 -> S/1
  world frame/1(Ang) -> Bus Creator/1
  world frame/2(AngVel) -> Bus Creator/2
  world frame/3(AngAccl1) -> Bus Creator/3
  world frame/4(LinPos1) -> Bus Creator/4
  world frame/5(LinVel1) -> Bus Creator/5
  world frame/6(LinAccl1) -> Bus Creator/6
  non rotating follower - vehicle frame/1(AngVehFrame) -> Bus Creator/7
  non rotating follower - vehicle frame/2(AngVelVehFrame) -> Bus Creator/8
  non rotating follower - vehicle frame/3(AngAcclVehFrame) -> Bus Creator/9
  non rotating follower - vehicle frame/4(LinPosVehFrame) -> Bus Creator/10
  non rotating follower - vehicle frame/5(LinVelVehFrame) -> Bus Creator/11
  non rotating follower - vehicle frame/6(LinAcclVehFrame) -> Bus Creator/12
  connections:
  non rotating follower - vehicle frame/LConn2 -- world frame/LConn2 -- World Frame/RConn1
  non rotating follower - vehicle frame/LConn1 -- world frame/LConn1 -- F/RConn1
